simulink library "adc"  (Simulink 8.1)
settings: Solver=ode45  StartTime=0.0  StopTime=10.0  RelTol=1e-3
undefined symbols (not defined in the file): ZERO_FLOAT
settings Model: Creator=AT015086  LastModifiedBy=tescamilla

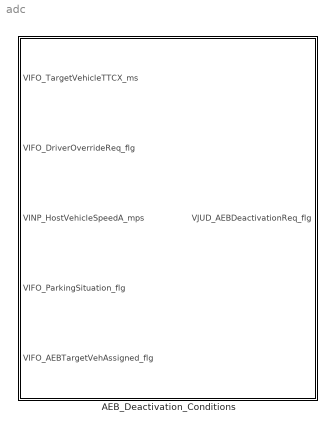
== system adc ==
  AEB_Deactivation_Conditions : Subsystem

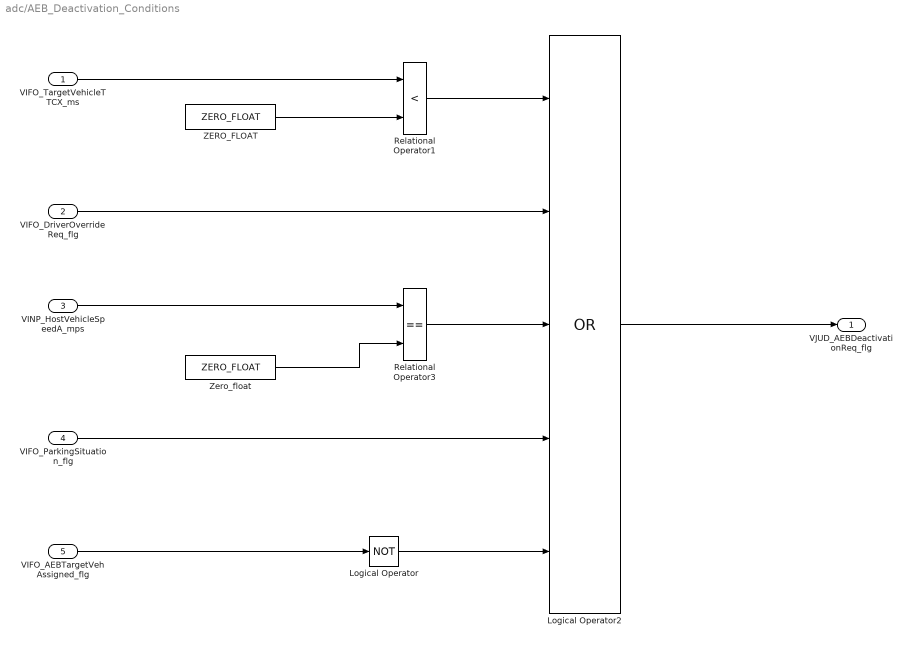
== system adc/AEB_Deactivation_Conditions ==
  VIFO_TargetVehicleTTCX_ms : Inport
  "VIFO_DriverOverrideReq_flg " : Inport  Port=2
  VINP_HostVehicleSpeedA_mps : Inport  Port=3
  VIFO_ParkingSituation_flg : Inport  Port=4
  VIFO_AEBTargetVehAssigned_flg : Inport  Port=5
  Logical Operator : Logic  Operator=NOT  AllPortsSameDT=off  OutDataTypeStr=boolean
  Logical Operator2 : Logic  Operator=OR  Inputs=5  AllPortsSameDT=off  OutDataTypeStr=boolean
  Relational Operator1 : RelationalOperator  Operator=<  OutDataTypeStr=boolean
  Relational Operator3 : RelationalOperator  Operator===  OutDataTypeStr=boolean
  ZERO_FLOAT : Constant  Value=ZERO_FLOAT
  Zero_float : Constant  Value=ZERO_FLOAT
  VJUD_AEBDeactivationReq_flg : Outport
  wires:
  VIFO_TargetVehicleTTCX_ms/1 -> Relational Operator1/1
  ZERO_FLOAT/1 -> Relational Operator1/2
  VINP_HostVehicleSpeedA_mps/1 -> Relational Operator3/1
  Zero_float/1 -> Relational Operator3/2
  "VIFO_DriverOverrideReq_flg "/1 -> Logical Operator2/2
  Logical Operator2/1 -> VJUD_AEBDeactivationReq_flg/1
  Relational Operator1/1 -> Logical Operator2/1
  Logical Operator/1 -> Logical Operator2/5
  Relational Operator3/1 -> Logical Operator2/3
  VIFO_ParkingSituation_flg/1 -> Logical Operator2/4
  VIFO_AEBTargetVehAssigned_flg/1 -> Logical Operator/1
